simulink model "interleaved_adc"  (R2024a)
settings: Solver=VariableStepAuto  StartTime=0.0  StopTime=5e-6  RelTol=1e-3  EnableMultiTasking=on
PostLoadFcn:
  | Fs_adc=1e9;  % Individual ADC sampling rate
InitFcn:
  | Fs_adc=1e9;  % Individual ADC sampling rate
libraries: dspfdesign x5, msbAdcMeasurements x1, commchan3 x1, simulink x1
settings Model: Creator=The MathWorks, Inc.  LastModifiedBy=Alexander
settings SolverCC: InitialStep=.1/1e9  AlgebraicLoopSolver=TrustRegion  MaxZcPerStep=1
settings DataIOCC: SaveFormat=Array  SaveOutput=off  SignalLogging=off  DSMLogging=off  SaveTime=off  ReturnWorkspaceOutputs=off  Refine=10
settings OptimizationCC: ExpressionDepthLimit=2147483647  InitFltsAndDblsToZero=on  LifeSpan=inf
settings DebuggingCC: SaveWithParameterizedLinksMsg=none  UnderspecifiedInitializationDetection=Classic  MergeDetectMultiDrivingBlocksExec=none  SignalResolutionControl=TryResolveAllWithWarning  SolverPrmCheckMsg=warning  MultiTaskDSMMsg=warning  MultiTaskCondExecSysMsg=none  IntegerOverflowMsg=none  ParameterOverflowMsg=none  ParameterPrecisionLossMsg=none  FcnCallInpInsideContextMsg=warning  UnconnectedInputMsg=warning  UnconnectedOutputMsg=warning  UnconnectedLineMsg=warning  StateNameClashWarn=warning  PregeneratedLibrarySubsystemCodeDiagnostic=none  SFUnexpectedBacktrackingDiag=warning  SFNoUnconditionalDefaultTransitionDiag=warning  SFExecutionAtInitializationDiag=none  IntegerSaturationMsg=none  ArithmeticOperatorsInVariantConditions=warning
settings HardwareCC: ProdBitPerPointer=32  ProdBitPerSizeT=32  ProdBitPerPtrDiffT=32  ProdLargestAtomicFloat=None  ProdIntDivRoundTo=Undefined  ProdEndianess=Unspecified  ProdWordSize=32  ProdHWDeviceType=32-bit Generic
settings ModelReferenceCC: EnableRefExpFcnMdlSchedulingChecks=on  PropagateSignalLabelsOutOfModel=off
settings SFSimCC: SimUseLocalCustomCode=off
settings RTWCC: RTWUseLocalCustomCode=off  BuildConfiguration=Faster Runs  GPUComputeCapability=3.5  DLArmComputeVersion=19.05
settings CodeAppCC: StateflowObjectComments=on
settings GRTTargetCC: TargetFcnLib=ansi_tfl_tmw.mat  TargetLangStandard=C89/C90 (ANSI)  CombineOutputUpdateFcns=off  GRTInterface=on
settings ConfigComp: CovMetricSettings=dw  CovSaveCumulativeToWorkspaceVar=on  CovSaveSingleToWorkspaceVar=on  CovExternalEMLEnable=off  CovSFcnEnable=off

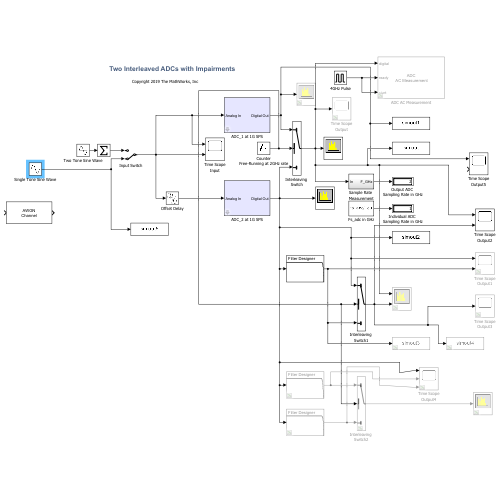
[thumbnail: Simulink's stored preview of the top-level diagram]
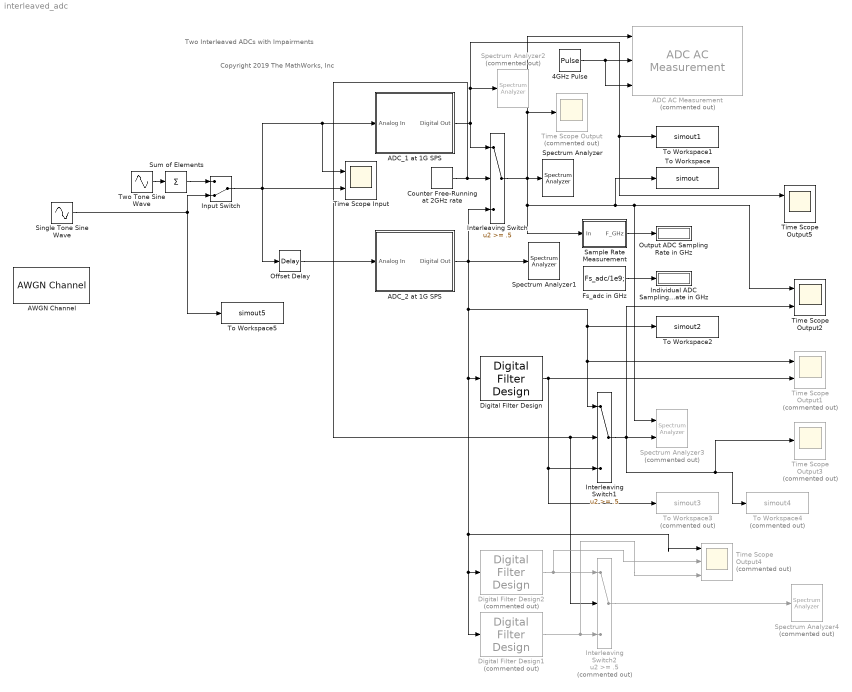
== system interleaved_adc ==
  note: Two Interleaved ADCs with Impairments
  note: Copyright 2019 The MathWorks, Inc
  4GHz Pulse : DiscretePulseGenerator  PulseType=Time based  Period="1  / (4 * Fs_adc)"  PulseWidth=50
  ADC AC Measurement : msbAdcMeasurements/ADC AC Measurement  Commented=on  DistortionMeasurement=Harmonic  InputFrequency=200e6  Method=Filter bank (slower, more precise, low leakage)  RBW=1953125  AutoSetRBW=on  NBits=5  Frequency=2 * 1e9  HoldOffTime=0  OutputToWorkspace=on  VariableName=interleaved_adc_output  ShowSpectrum=off
  ADC_1 at 1G SPS : Subsystem  mask{Fadc=Fs_adc, jitter=off, nonlinearity=off, quantization=off, seed=123}
      mask prompts: Fadc "ADC sample rate (Hz)"; jitter "Enable jitter"; nonlinearity "Enable non-linearity"; quantization "Enable quantization and saturation"; seed "Noise seed"
      mask DialogControl DescGroupVar Prompt: ADC
      mask DialogControl DescTextVar Prompt: Simple ADC model with tunable impairments
  ADC_2 at 1G SPS : Subsystem  mask{Fadc=Fs_adc, jitter=off, nonlinearity=off, quantization=off, seed=345}
      mask prompts: Fadc "ADC sample rate (Hz)"; jitter "Enable jitter"; nonlinearity "Enable non-linearity"; quantization "Enable quantization and saturation"; seed "Noise seed"
      mask DialogControl DescGroupVar Prompt: ADC
      mask DialogControl DescTextVar Prompt: Simple ADC model with tunable impairments
  AWGN Channel : commchan3/AWGN Channel  LegacyMode=off  NoiseMethod="Signal to noise ratio  (SNR)"  noiseMode="Signal to noise ratio  (SNR)"  EbNo=10  EsNo=10  SNR=62  BitsPerSymbol=1  SignalPower=1  SamplesPerSymbol=1  SymbolPeriod=1  VarianceSource=Parameter  Variance=1  RandomStream=Global stream  Seed=67  SimulateUsing=Code generation
  Counter Free-Running at 2GHz rate : simulink/Sources/Counter Free-Running  NumBits=1  tsamp=.5/Fs_adc
  Digital Filter Design : dspfdesign/Digital Filter Design  mwdsp_browser_bugfix_var=off
  Digital Filter Design1 : dspfdesign/Digital Filter Design  Commented=on  mwdsp_browser_bugfix_var=off
  Digital Filter Design2 : dspfdesign/Digital Filter Design  Commented=on  mwdsp_browser_bugfix_var=off
  Fs_adc in GHz : Constant  Value=Fs_adc/1e9;
  Individual ADC Sampling Rate in GHz : Display
  Input Switch : ManualSwitch  CurrentSetting=0
  Interleaving Switch : Switch  Threshold=.5  SaturateOnIntegerOverflow=off  InputSameDT=off
  Interleaving Switch1 : Switch  Threshold=.5  SaturateOnIntegerOverflow=off  InputSameDT=off
  Interleaving Switch2 : Switch  Commented=on  Threshold=.5  SaturateOnIntegerOverflow=off  InputSameDT=off
  Offset Delay : TransportDelay  DelayTime=.5/Fs_adc
  Output ADC Sampling Rate in GHz : Display
      settings: Decimation=1000
  Sample Rate Measurement : Subsystem
  Single Tone Sine Wave : Sin  Amplitude=.5*1.2  Frequency=2*pi*[40]*1e6  SampleTime=0
  Spectrum Analyzer : SpectrumAnalyzer  WindowPosition=[2.000000,37.000000,2556.000000,1366.000000,]  Visible=on  ScopeFrameLocation=window  Method=Welch  SampleRate=2000000000  PlotAsTwoSidedSpectrum=off  AxesScaling=Manual  FrequencyResolutionMethod=Window length  WindowLength=2048  FFTLengthSource=Property  FFTLength=2048  Span=1000000000  CenterFrequency=500000000  StartFrequency=0  StopFrequency=1000000000  AveragingMethod=Running  SpectralAverages=2  YLabel=Magnitude-squared  YLimits=[-326.84077069,59.61464133]  SelectedToolstripTab=spectrumAnalyzerToolstrip.measurementsTab  AllowFFTLengthLessThanSamplesPerUpdate=on  DefaultConfigurationName=spbscopes.SpectrumAnalyzerBlockCfg  IsFrequencyInputMode=0  FrequencyVectorPort=0  FrequencyVectorFromPort=0  FrequencyInputRBWPort=0  FrequencyInputRBWFromPort=0  SegLen=2048
  Spectrum Analyzer1 : SpectrumAnalyzer  WindowPosition=[2.000000,37.000000,2556.000000,1366.000000,]  Visible=on  ScopeFrameLocation=window  Method=Welch  SampleRate=2000000000  PlotAsTwoSidedSpectrum=off  AxesScaling=Manual  FrequencyResolutionMethod=Window length  WindowLength=2048  FFTLengthSource=Property  FFTLength=2048  Span=1000000000  CenterFrequency=500000000  StartFrequency=0  StopFrequency=1000000000  AveragingMethod=Running  SpectralAverages=2  YLabel=Magnitude-squared  YLimits=[-326.84077069,59.61464133]  SelectedToolstripTab=spectrumAnalyzerToolstrip.measurementsTab  AllowFFTLengthLessThanSamplesPerUpdate=on  DefaultConfigurationName=spbscopes.SpectrumAnalyzerBlockCfg  IsFrequencyInputMode=0  FrequencyVectorPort=0  FrequencyVectorFromPort=0  FrequencyInputRBWPort=0  FrequencyInputRBWFromPort=0  SegLen=2048
  Spectrum Analyzer2 : SpectrumAnalyzer  Commented=on  WindowPosition=[0.000000,32.000000,2560.000000,1376.000000,]  ScopeFrameLocation=window  Method=Welch  SampleRate=2000000000  PlotAsTwoSidedSpectrum=off  AxesScaling=Manual  FrequencyResolutionMethod=Window length  WindowLength=2048  FFTLengthSource=Property  FFTLength=2048  Span=1000000000  CenterFrequency=500000000  StartFrequency=0  StopFrequency=1000000000  AveragingMethod=Running  SpectralAverages=2  YLabel=Magnitude-squared  YLimits=[-326.84077069,59.61464133]  SelectedToolstripTab=spectrumAnalyzerToolstrip.measurementsTab  AllowFFTLengthLessThanSamplesPerUpdate=on  DefaultConfigurationName=spbscopes.SpectrumAnalyzerBlockCfg  IsFrequencyInputMode=0  FrequencyVectorPort=0  FrequencyVectorFromPort=0  FrequencyInputRBWPort=0  FrequencyInputRBWFromPort=0  SegLen=2048
  Spectrum Analyzer3 : SpectrumAnalyzer  Commented=on  NumInputPorts=2  WindowPosition=[2.000000,40.000000,2556.000000,1361.000000,]  ScopeFrameLocation=window  Method=Welch  SampleRate=2000000000  PlotAsTwoSidedSpectrum=off  AxesScaling=Manual  FrequencyResolutionMethod=Window length  WindowLength=2048  FFTLengthSource=Property  FFTLength=2048  Span=1000000000  CenterFrequency=500000000  StartFrequency=0  StopFrequency=1000000000  AveragingMethod=Running  SpectralAverages=2  YLabel=Magnitude-squared  YLimits=[-99.85959046,35.14786912]  ExpandToolstrip=on  SelectedToolstripTab=spectrumAnalyzerToolstrip.measurementsTab  MeasurementChannel=2  AllowFFTLengthLessThanSamplesPerUpdate=on  DefaultConfigurationName=spbscopes.SpectrumAnalyzerBlockCfg  IsFrequencyInputMode=0  FrequencyVectorPort=0  FrequencyVectorFromPort=0  FrequencyInputRBWPort=0  FrequencyInputRBWFromPort=0  SegLen=2048
  Spectrum Analyzer4 : SpectrumAnalyzer  Commented=on  WindowPosition=[2.000000,37.000000,2556.000000,1366.000000,]  ScopeFrameLocation=window  Method=Welch  SampleRate=2000000000  PlotAsTwoSidedSpectrum=off  AxesScaling=Manual  FrequencyResolutionMethod=Window length  WindowLength=2048  FFTLengthSource=Property  FFTLength=2048  Span=1000000000  CenterFrequency=500000000  StartFrequency=0  StopFrequency=1000000000  AveragingMethod=Running  SpectralAverages=2  YLabel=Magnitude-squared  YLimits=[-326.84077069,59.61464133]  SelectedToolstripTab=spectrumAnalyzerToolstrip.measurementsTab  AllowFFTLengthLessThanSamplesPerUpdate=on  DefaultConfigurationName=spbscopes.SpectrumAnalyzerBlockCfg  IsFrequencyInputMode=0  FrequencyVectorPort=0  FrequencyVectorFromPort=0  FrequencyInputRBWPort=0  FrequencyInputRBWFromPort=0  SegLen=2048
  Sum of Elements : Sum  Inputs=+
  Time Scope Input : Scope  NumInputPorts=2
  Time Scope Output : Scope  Commented=on
  Time Scope Output1 : Scope  Commented=on  NumInputPorts=2
  Time Scope Output2 : Scope  NumInputPorts=2
  Time Scope Output3 : Scope  Commented=on
  Time Scope Output4 : Scope  Commented=on  NumInputPorts=3
  Time Scope Output5 : Scope  NumInputPorts=2
  To Workspace : ToWorkspace  VariableName=simout  SampleTime=-1
      settings: Save2DSignal=2-D array (concatenate along first dimension)
  To Workspace1 : ToWorkspace  VariableName=simout1  SampleTime=-1
      settings: Save2DSignal=2-D array (concatenate along first dimension)
  To Workspace2 : ToWorkspace  VariableName=simout2  SampleTime=-1
      settings: Save2DSignal=2-D array (concatenate along first dimension)
  To Workspace3 : ToWorkspace  Commented=on  VariableName=simout3  SampleTime=-1
      settings: Save2DSignal=2-D array (concatenate along first dimension)
  To Workspace4 : ToWorkspace  Commented=on  VariableName=simout4  SampleTime=-1
      settings: Save2DSignal=2-D array (concatenate along first dimension)
  To Workspace5 : ToWorkspace  VariableName=simout5  SampleTime=-1
      settings: Save2DSignal=2-D array (concatenate along first dimension)
  Two Tone Sine Wave : Sin  Amplitude=.5  Frequency=2*pi*[203.125, 218.750]*1e6  SampleTime=0
  wires:
  Two Tone Sine Wave/1 -> Sum of Elements/1
  Input Switch/1 -> Time Scope Input/1, ADC_1 at 1G SPS/1(Analog In), Offset Delay/1, Time Scope Input/2
  Counter Free-Running at 2GHz rate/1 -> Interleaving Switch2/2, Interleaving Switch1/2, Interleaving Switch/2
  Interleaving Switch/1 -> Spectrum Analyzer/1, Sample Rate Measurement/1(In), Time Scope Output2/1, Spectrum Analyzer3/1, To Workspace/1, ADC AC Measurement/1, Time Scope Output/1
  ADC_2 at 1G SPS/1(Digital Out) -> Interleaving Switch/3, Spectrum Analyzer1/1, Time Scope Output4/1, Digital Filter Design1/1, Digital Filter Design2/1, Digital Filter Design/1, Time Scope Output1/1, Interleaving Switch1/1, To Workspace2/1
  ADC_1 at 1G SPS/1(Digital Out) -> Time Scope Output5/1, To Workspace1/1, Spectrum Analyzer2/1, Interleaving Switch/1
  Fs_adc in GHz/1 -> Individual ADC Sampling Rate in GHz/1
  Sample Rate Measurement/1(F_GHz) -> Output ADC Sampling Rate in GHz/1
  4GHz Pulse/1 -> ADC AC Measurement/2, ADC AC Measurement/3
  Sum of Elements/1 -> Input Switch/1
  Interleaving Switch1/1 -> Time Scope Output3/1, To Workspace4/1, Spectrum Analyzer3/2, Time Scope Output2/2
  Digital Filter Design/1 -> Time Scope Output1/2, To Workspace3/1, Interleaving Switch1/3
  Digital Filter Design2/1 -> Time Scope Output4/2, Interleaving Switch2/1
  Digital Filter Design1/1 -> Time Scope Output4/3, Interleaving Switch2/3
  Interleaving Switch2/1 -> Spectrum Analyzer4/1
  Offset Delay/1 -> ADC_2 at 1G SPS/1(Analog In)
  Single Tone Sine Wave/1 -> To Workspace5/1, Input Switch/2

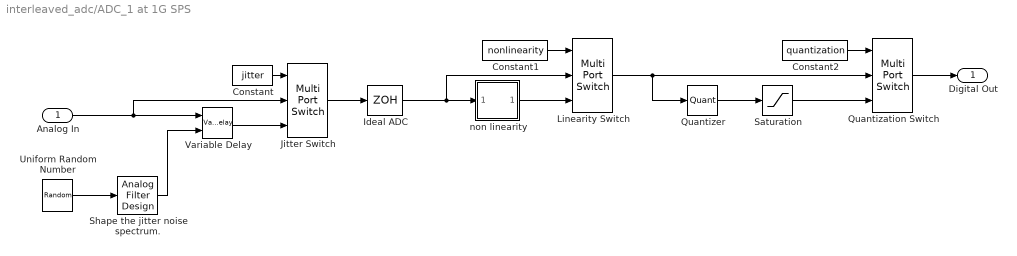
== system interleaved_adc/ADC_1 at 1G SPS ==
  Analog In : Inport
  Constant : Constant  Value=jitter
  Constant1 : Constant  Value=nonlinearity
  Constant2 : Constant  Value=quantization
  Ideal ADC : ZeroOrderHold  SampleTime=1/Fadc
  "Jitter Switch " : MultiPortSwitch  DataPortOrder=Zero-based contiguous  Inputs=2  zeroidx=on  SaturateOnIntegerOverflow=off  InputSameDT=off
  Linearity Switch : MultiPortSwitch  DataPortOrder=Zero-based contiguous  Inputs=2  zeroidx=on  SaturateOnIntegerOverflow=off  InputSameDT=off
  Quantization Switch : MultiPortSwitch  DataPortOrder=Zero-based contiguous  Inputs=2  zeroidx=on  SaturateOnIntegerOverflow=off  InputSameDT=off
  Quantizer : Quantizer  QuantizationInterval=2^-8
  Saturation : Saturate  UpperLimit=1  LowerLimit=-1
  "Shape the jitter noise spectrum. " : dspfdesign/Analog Filter Design  method=Butterworth  filttype=Lowpass  N=3  Wlo=2*pi*40e6  Whi=80  Rp=2  Rs=40
  Uniform Random Number : UniformRandomNumber  Minimum=0  Maximum=0.5e-9  Seed=seed  SampleTime=.1/40e6
  Variable Delay : VariableTransportDelay  MaximumDelay=3e-9  ZeroDelay=on  TransDelayFeedthrough=on
  non linearity : Subsystem  mask{alpha=.2}
      mask init:
      | x=-3:0.01:3;  y= (1/alpha)*tanh(alpha*x) ;
      mask Display: plot(x,y)
  Digital Out : Outport  VectorParamsAs1DForOutWhenUnconnected=off
  wires:
  Uniform Random Number/1 -> "Shape the jitter noise spectrum. "/1
  Quantizer/1 -> Saturation/1
  "Shape the jitter noise spectrum. "/1 -> Variable Delay/2
  Ideal ADC/1 -> Linearity Switch/2, non linearity/1(In1)
  Linearity Switch/1 -> Quantization Switch/2, Quantizer/1
  Quantization Switch/1 -> Digital Out/1
  "Jitter Switch "/1 -> Ideal ADC/1
  Variable Delay/1 -> "Jitter Switch "/3
  Analog In/1 -> "Jitter Switch "/2, Variable Delay/1
  non linearity/1(Out1) -> Linearity Switch/3
  Saturation/1 -> Quantization Switch/3
  Constant/1 -> "Jitter Switch "/1
  Constant1/1 -> Linearity Switch/1
  Constant2/1 -> Quantization Switch/1

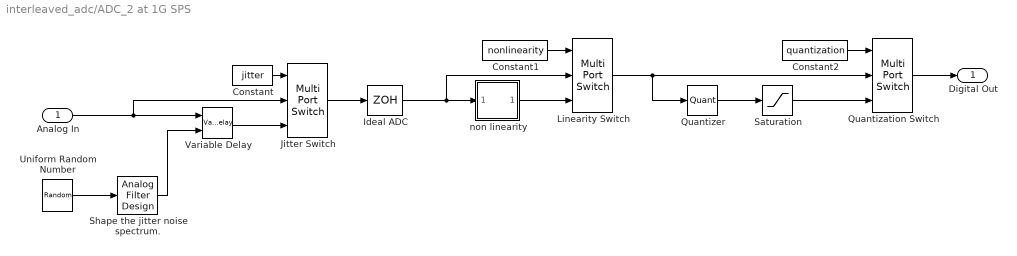
== system interleaved_adc/ADC_2 at 1G SPS ==
  Analog In : Inport
  Constant : Constant  Value=jitter
  Constant1 : Constant  Value=nonlinearity
  Constant2 : Constant  Value=quantization
  Ideal ADC : ZeroOrderHold  SampleTime=1/Fadc
  "Jitter Switch " : MultiPortSwitch  DataPortOrder=Zero-based contiguous  Inputs=2  zeroidx=on  SaturateOnIntegerOverflow=off  InputSameDT=off
  Linearity Switch : MultiPortSwitch  DataPortOrder=Zero-based contiguous  Inputs=2  zeroidx=on  SaturateOnIntegerOverflow=off  InputSameDT=off
  Quantization Switch : MultiPortSwitch  DataPortOrder=Zero-based contiguous  Inputs=2  zeroidx=on  SaturateOnIntegerOverflow=off  InputSameDT=off
  Quantizer : Quantizer  QuantizationInterval=2^-8
  Saturation : Saturate  UpperLimit=1  LowerLimit=-1
  "Shape the jitter noise spectrum. " : dspfdesign/Analog Filter Design  method=Butterworth  filttype=Lowpass  N=3  Wlo=2*pi*40e6  Whi=80  Rp=2  Rs=40
  Uniform Random Number : UniformRandomNumber  Minimum=0  Maximum=0.5e-9  Seed=seed  SampleTime=.1/40e6
  Variable Delay : VariableTransportDelay  MaximumDelay=3e-9  ZeroDelay=on  TransDelayFeedthrough=on
  non linearity : Subsystem  mask{alpha=.2}
      mask init:
      | x=-3:0.01:3;  y= (1/alpha)*tanh(alpha*x) ;
      mask Display: plot(x,y)
  Digital Out : Outport  VectorParamsAs1DForOutWhenUnconnected=off
  wires:
  Constant2/1 -> Quantization Switch/1
  Constant1/1 -> Linearity Switch/1
  Constant/1 -> "Jitter Switch "/1
  Saturation/1 -> Quantization Switch/3
  non linearity/1(Out1) -> Linearity Switch/3
  Analog In/1 -> Variable Delay/1, "Jitter Switch "/2
  Variable Delay/1 -> "Jitter Switch "/3
  "Jitter Switch "/1 -> Ideal ADC/1
  Quantization Switch/1 -> Digital Out/1
  Linearity Switch/1 -> Quantizer/1, Quantization Switch/2
  Ideal ADC/1 -> non linearity/1(In1), Linearity Switch/2
  "Shape the jitter noise spectrum. "/1 -> Variable Delay/2
  Quantizer/1 -> Saturation/1
  Uniform Random Number/1 -> "Shape the jitter noise spectrum. "/1

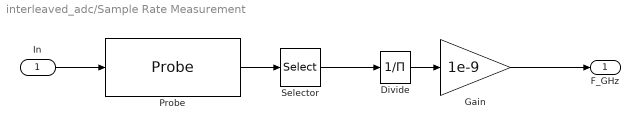
== system interleaved_adc/Sample Rate Measurement ==
  In : Inport
  Divide : Product  Inputs=/
  Gain : Gain  Gain=1e-9
  Probe : Probe  ProbeWidth=off  ProbeComplexSignal=off
  Selector : Selector  InputPortWidth=2  IndexOptions=Index vector (dialog)  Indices=1  OutputSizes=1
  F_GHz : Outport  VectorParamsAs1DForOutWhenUnconnected=off
  wires:
  Gain/1 -> F_GHz/1
  Probe/1 -> Selector/1
  Selector/1 -> Divide/1
  Divide/1 -> Gain/1
  In/1 -> Probe/1

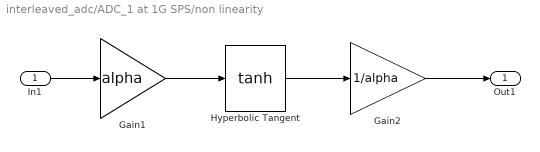
== system interleaved_adc/ADC_1 at 1G SPS/non linearity ==
  In1 : Inport
  Gain1 : Gain  Gain=alpha  SaturateOnIntegerOverflow=on  OutDataTypeStr=Inherit: Same as input  ParamDataTypeStr=Inherit: Same as input
  Gain2 : Gain  Gain=1/alpha  SaturateOnIntegerOverflow=on  OutDataTypeStr=Inherit: Same as input  ParamDataTypeStr=Inherit: Same as input
  Hyperbolic Tangent : Trigonometry  Operator=tanh
  Out1 : Outport  VectorParamsAs1DForOutWhenUnconnected=off
  wires:
  Hyperbolic Tangent/1 -> Gain2/1
  In1/1 -> Gain1/1
  Gain2/1 -> Out1/1
  Gain1/1 -> Hyperbolic Tangent/1

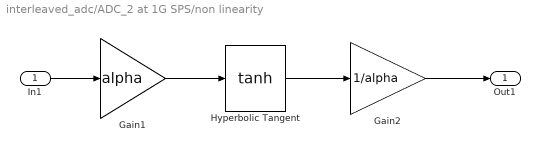
== system interleaved_adc/ADC_2 at 1G SPS/non linearity ==
  In1 : Inport
  Gain1 : Gain  Gain=alpha  SaturateOnIntegerOverflow=on  OutDataTypeStr=Inherit: Same as input  ParamDataTypeStr=Inherit: Same as input
  Gain2 : Gain  Gain=1/alpha  SaturateOnIntegerOverflow=on  OutDataTypeStr=Inherit: Same as input  ParamDataTypeStr=Inherit: Same as input
  Hyperbolic Tangent : Trigonometry  Operator=tanh
  Out1 : Outport  VectorParamsAs1DForOutWhenUnconnected=off
  wires:
  Gain1/1 -> Hyperbolic Tangent/1
  Gain2/1 -> Out1/1
  In1/1 -> Gain1/1
  Hyperbolic Tangent/1 -> Gain2/1
